simulink model "flybackConverter"  (R2023a)
settings: Solver=ode23t  StartTime=0.0  StopTime=1  MaxStep=1e-4  RelTol=1e-3
model workspace (MAT data in the model file):
  C = Simulink.Parameter
  C.Value = 0.0001
  C.DataType = 'auto'
  C.Complexity = 'real'
  C.Dimensions = [1 1]
  Fs = Simulink.Parameter
  Fs.Value = 1000000
  Fs.DataType = 'auto'
  Fs.Complexity = 'real'
  Fs.Dimensions = [1 1]
  Lm = Simulink.Parameter
  Lm.Value = 0.01
  Lm.DataType = 'auto'
  Lm.Complexity = 'real'
  Lm.Dimensions = [1 1]
  N1 = Simulink.Parameter
  N1.Value = 100
  N1.DataType = 'auto'
  N1.Complexity = 'real'
  N1.Dimensions = [1 1]
  N2 = Simulink.Parameter
  N2.Value = 100
  N2.DataType = 'auto'
  N2.Complexity = 'real'
  N2.Dimensions = [1 1]
  R = Simulink.Parameter
  R.Value = 10
  R.DataType = 'auto'
  R.Complexity = 'real'
  R.Dimensions = [1 1]
  Vin = Simulink.Parameter
  Vin.Value = 24
  Vin.DataType = 'auto'
  Vin.Complexity = 'real'
  Vin.Dimensions = [1 1]
libraries: spsSeriesRLCBranchLib x4, spsVoltageMeasurementLib x3, spsCurrentMeasurementLib x2, spsDCVoltageSourceLib x1, spsDiodeLib x1, spsIGBTDiodeLib x1, spsLinearTransformerLib x1, spsMeanLib x1, spsRMSLib x1, spspowerguiLib x1
settings Model: Creator=User  LastModifiedBy=User
settings SolverCC: ZeroCrossAlgorithm=Adaptive
settings DebuggingCC: IgnoredZcDiagnostic=none  UnconnectedInputMsg=warning  UnconnectedOutputMsg=warning  UnconnectedLineMsg=warning
settings ModelReferenceCC: EnableRefExpFcnMdlSchedulingChecks=on
settings RTWCC: DLArmComputeVersion=19.05

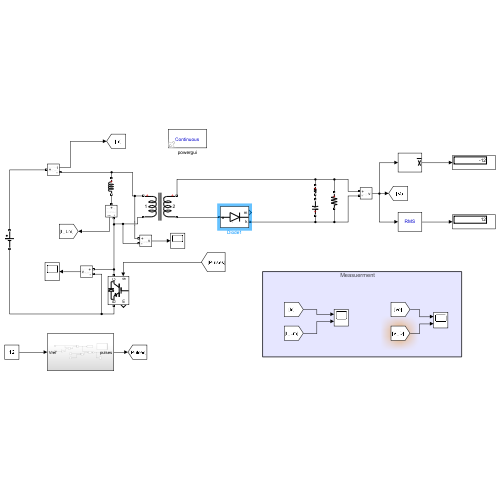
[thumbnail: Simulink's stored preview of the top-level diagram]
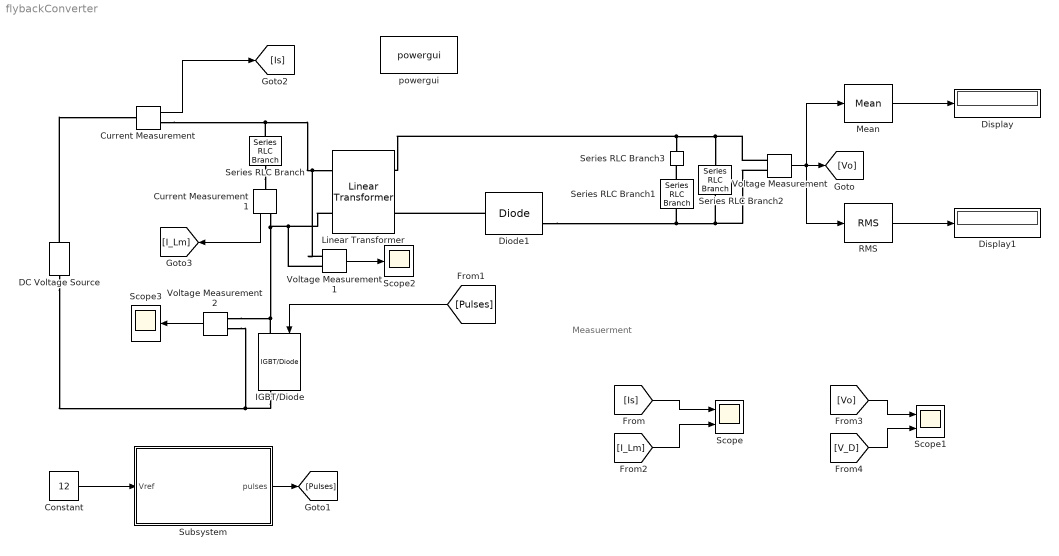
== system flybackConverter ==
  note: Measuerment
  Constant : Constant  Value=12
  Current Measurement : spsCurrentMeasurementLib/Current Measurement  PhasorSimulation=off  OutputType=Complex  PSBequivalent=0
  Current Measurement1 : spsCurrentMeasurementLib/Current Measurement  PhasorSimulation=off  OutputType=Complex  PSBequivalent=0
  DC Voltage Source : spsDCVoltageSourceLib/DC Voltage Source  Amplitude=Vin  Measurements=None
  Diode1 : spsDiodeLib/Diode  Ron=0.001  Lon=0  Vf=0.8  IC=0  UseSnubber=0  Rs=500  Cs=250e-9  Measurements=on
  Display : Display
  Display1 : Display
  IGBT/Diode : spsIGBTDiodeLib/IGBT//Diode  Ron=1e-3  Rs=1e5  Cs=inf  Measurements=on
  Linear Transformer : spsLinearTransformerLib/Linear Transformer  UNITS=pu  NominalPower=[ 3000 5000 ]  winding1="[ N1  0  0 ]"  winding2="[ N2  0  0 ]"  ThreeWindings=off  winding3=[ 315e3 0.002 0.08 ]  RmLm=[ 500 500 ]  Measurements=None  DataType=off
  Mean : spsMeanLib/Mean  Freq=60  Vinit=0  Ts=0
  RMS : spsRMSLib/RMS  TrueRMS=on  Freq=60  RMSInit=120  Ts=0
  Scope : Scope  NumInputPorts=2
  Scope1 : Scope  NumInputPorts=2
  Scope2 : Scope
  Scope3 : Scope
  Series RLC Branch : spsSeriesRLCBranchLib/Series RLC Branch  LConnTagsString=__new0  RConnTagsString=__new0  BranchType=L  Resistance=1  Inductance=Lm  SetiL0=off  InitialCurrent=0  Capacitance=1e-6  Setx0=off  InitialVoltage=0  Measurements=None
  Series RLC Branch1 : spsSeriesRLCBranchLib/Series RLC Branch  LConnTagsString=__new0  RConnTagsString=__new0  BranchType=C  Resistance=1  Inductance=1e-3  SetiL0=off  InitialCurrent=0  Capacitance=C  Setx0=off  InitialVoltage=0  Measurements=None
  Series RLC Branch2 : spsSeriesRLCBranchLib/Series RLC Branch  LConnTagsString=__new0  RConnTagsString=__new0  BranchType=R  Resistance=R  Inductance=1e-3  SetiL0=off  InitialCurrent=0  Capacitance=1e-6  Setx0=off  InitialVoltage=0  Measurements=None
  Series RLC Branch3 : spsSeriesRLCBranchLib/Series RLC Branch  LConnTagsString=__new0  RConnTagsString=__new0  BranchType=R  Resistance=.000001  Inductance=1e-3  SetiL0=off  InitialCurrent=0  Capacitance=1e-6  Setx0=off  InitialVoltage=0  Measurements=None
  Subsystem : Subsystem
  Voltage Measurement : spsVoltageMeasurementLib/Voltage Measurement  PhasorSimulation=off  OutputType=Complex  PSBequivalent=0
  Voltage Measurement1 : spsVoltageMeasurementLib/Voltage Measurement  PhasorSimulation=off  OutputType=Complex  PSBequivalent=0
  Voltage Measurement2 : spsVoltageMeasurementLib/Voltage Measurement  PhasorSimulation=off  OutputType=Complex  PSBequivalent=0
  powergui : spspowerguiLib/powergui  Priority=1  SimulationMode=Continuous  SampleTime=50e-6  frequency=60  Iterations=50  frequencyindice=0  Pbase=100e6  ErrMax=1e-4  UnitsV=kV  UnitsW=MW  buscounter=0  FunctionMessages=off  echomessages=off  EnableUseOfTLC=off  CurrentSourceSwitches=off  DisableSnubberDevices=on  DisableRonSwitches=on  DisableVfSwitches=on  DisplayEquations=on  AutomaticDiscreteSolvers=off  SolverType=Tustin/Backward Euler (TBE)  Interpol=off  ExternalGateDelay=off  methode=off  Ts=100  x0status=blocks  SPID=on  SwTol=0  HookPort=off  NonlinearTolerance=1e-4  nMaxIteration=100  ContinueOnMaxIteration=off  RestoreLinks=warning  ResistiveCurrentMeasurement=off  Frange=[0:2:500]  Ylog=off  Xlog=on  ShowGrid=off  save=off  variable=ZData  structure=0  ZoomFFT=off  StartTime=0.0  cycles=1  DisplayStyle=1  fundamental=60  FreqAxis=off  MaxFrequency=1000  frequencyindicesteady=1  RmsSteady=1  display=off
  wires:
  Voltage Measurement/1 -> Mean/1, RMS/1, [Vo]
  Subsystem/1(pulses) -> [Pulses]
  Current Measurement/1 -> [Is]
  Current Measurement1/1 -> [I_Lm]
  [Is] -> Scope/1
  [I_Lm] -> Scope/2
  [Vo] -> Scope1/1
  [V_D] -> Scope1/2
  Constant/1 -> Subsystem/1(Vref)
  Mean/1 -> Display/1
  RMS/1 -> Display1/1
  [Pulses] -> IGBT/Diode/1
  Voltage Measurement1/1 -> Scope2/1
  Voltage Measurement2/1 -> Scope3/1
  connections:
  DC Voltage Source/LConn1 -- IGBT/Diode/RConn1 -- Voltage Measurement2/LConn2
  Series RLC Branch/RConn1 -- Current Measurement1/LConn1
  Current Measurement/RConn1 -- Series RLC Branch/LConn1 -- Voltage Measurement1/LConn1 -- Linear Transformer/LConn1
  Voltage Measurement/LConn2 -- Diode1/RConn1 -- Series RLC Branch1/LConn1 -- Series RLC Branch2/RConn1
  DC Voltage Source/RConn1 -- Current Measurement/LConn1
  Linear Transformer/LConn2 -- Voltage Measurement1/LConn2 -- Current Measurement1/RConn1 -- IGBT/Diode/LConn1 -- Voltage Measurement2/LConn1
  Voltage Measurement/LConn1 -- Linear Transformer/RConn1 -- Series RLC Branch3/LConn1 -- Series RLC Branch2/LConn1
  Series RLC Branch1/RConn1 -- Series RLC Branch3/RConn1
  Diode1/LConn1 -- Linear Transformer/RConn2

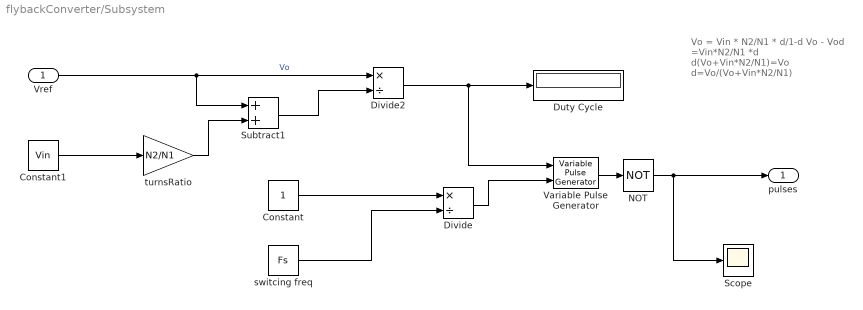
== system flybackConverter/Subsystem ==
  note: Vo = Vin * N2/N1 * d/1-d
      |
      | Vo - Vod =Vin*N2/N1 *d
      |
      | d(Vo+Vin*N2/N1)=Vo
      |
      | d=Vo/(Vo+Vin*N2/N1)
  Vref : Inport
  Constant : Constant
  Constant1 : Constant  Value=Vin
  Divide : Product  Inputs=*/
  Divide2 : Product  Inputs=*/
  Duty Cycle : Display
  NOT : Logic  Operator=NOT  IconShape=distinctive  AllPortsSameDT=off  OutDataTypeStr=boolean
  Scope : Scope
  Subtract1 : Sum
  Variable Pulse Generator : VariablePulseGenerator  AllowZeroPulseWidth=on  SampleTime=0.1
  switcing freq : Constant  Value=Fs
  turnsRatio : Gain  Gain=N2/N1
  pulses : Outport
  wires:
  Divide/1 -> Variable Pulse Generator/2
  Vref/1 -> Divide2/1, Subtract1/1  "Vo"
  Constant1/1 -> turnsRatio/1
  turnsRatio/1 -> Subtract1/2
  Subtract1/1 -> Divide2/2
  Constant/1 -> Divide/1
  switcing freq/1 -> Divide/2
  Divide2/1 -> Variable Pulse Generator/1, Duty Cycle/1
  Variable Pulse Generator/1 -> NOT/1
  NOT/1 -> Scope/1, pulses/1
